simulink model "delayed_output"  (R2023b)
settings: Solver=VariableStepAuto  StartTime=0.0  StopTime=10.0  FixedStep=0.002  RelTol=1e-3
libraries: simulink x1
settings Model: Creator=franc  LastModifiedBy=franc

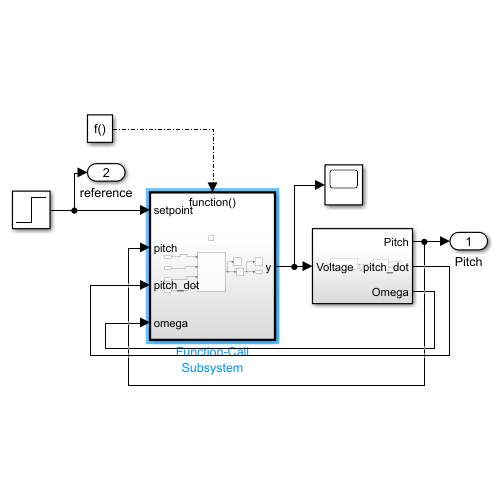
[thumbnail: Simulink's stored preview of the top-level diagram]
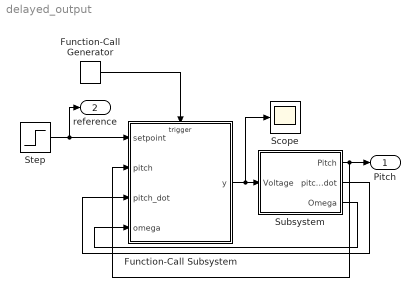
== system delayed_output ==
  Function-Call Generator : simulink/Ports & Subsystems/Function-Call Generator  sample_time=0.1  numberOfIterations=1  DisallowWideOutput=off
  Function-Call Subsystem : Subsystem  TreatAsAtomicUnit=on
  Scope : Scope
  Step : Step  SampleTime=0
  Subsystem : Subsystem
  Pitch : Outport
  reference : Outport  Port=2
  wires:
  Function-Call Generator/1 -> Function-Call Subsystem/Trigger
  Step/1 -> reference/1, Function-Call Subsystem/1(setpoint)
  Function-Call Subsystem/1(y) -> Scope/1, Subsystem/1(Voltage)
  Subsystem/2(pitch_dot) -> Function-Call Subsystem/3(pitch_dot)
  Subsystem/3(Omega) -> Function-Call Subsystem/4(omega)
  Subsystem/1(Pitch) -> Pitch/1, Function-Call Subsystem/2(pitch)

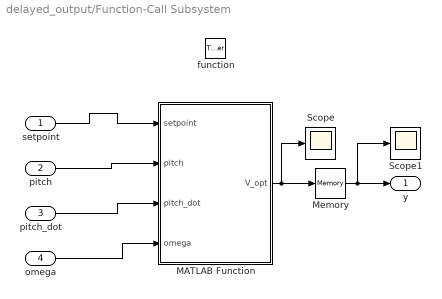
== system delayed_output/Function-Call Subsystem ==
  setpoint : Inport
  pitch : Inport  Port=2
  pitch_dot : Inport  Port=3
  omega : Inport  Port=4
  function : TriggerPort  TriggerType=function-call  VariantControl=(inherit)  SampleTimeType=periodic  SampleTime=0.1
  MATLAB Function : MATLAB Function  TreatAsAtomicUnit=on
  Memory : Memory  InheritSampleTime=on
  Scope : Scope
  Scope1 : Scope
  y : Outport
  wires:
  setpoint/1 -> MATLAB Function/1(setpoint)
  MATLAB Function/1(V_opt) -> Scope/1, Memory/1
  pitch/1 -> MATLAB Function/2(pitch)
  pitch_dot/1 -> MATLAB Function/3(pitch_dot)
  omega/1 -> MATLAB Function/4(omega)
  Memory/1 -> Scope1/1, y/1

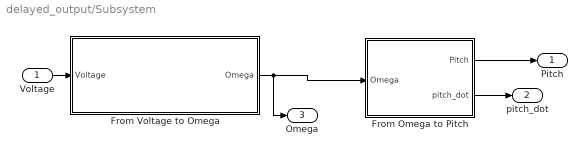
== system delayed_output/Subsystem ==
  Voltage : Inport
  From Omega to Pitch : Subsystem
  From Voltage to Omega : Subsystem
  Pitch : Outport
  pitch_dot : Outport  Port=2
  Omega : Outport  Port=3
  wires:
  From Voltage to Omega/1(Omega) -> Omega/1, From Omega to Pitch/1(Omega)
  Voltage/1 -> From Voltage to Omega/1(Voltage)
  From Omega to Pitch/1(Pitch) -> Pitch/1
  From Omega to Pitch/2(pitch_dot) -> pitch_dot/1

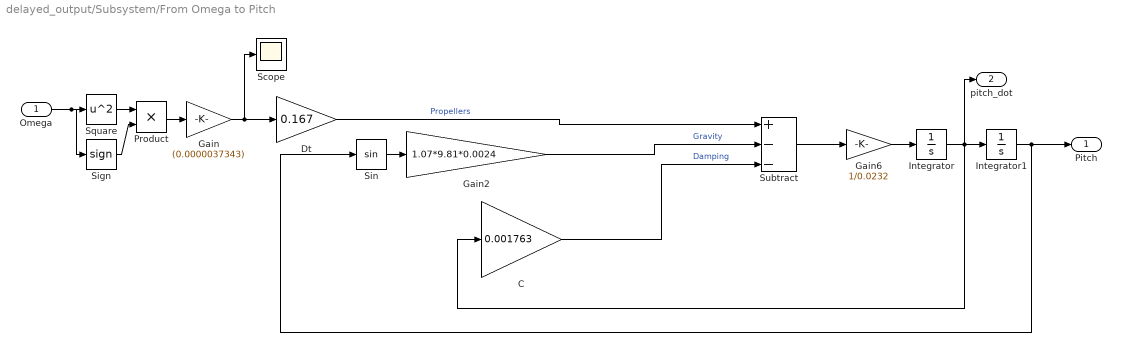
== system delayed_output/Subsystem/From Omega to Pitch ==
  Omega : Inport
  C : Gain  Gain=0.001763
  Dt : Gain  Gain=0.167
  Gain : Gain  Gain=(0.0000037343)
  Gain2 : Gain  Gain=1.07*9.81*0.0024
  Gain6 : Gain  Gain=1/0.0232
  Integrator : Integrator
  Integrator1 : Integrator
  Product : Product
  Scope : Scope
  Sign : Signum  ZeroCross=off
  Sin : Trigonometry
  Square : Math  Operator=square
  Subtract : Sum  Inputs=+--
  Pitch : Outport
  pitch_dot : Outport  Port=2
  wires:
  Integrator1/1 -> Pitch/1, Sin/1
  Sin/1 -> Gain2/1
  Subtract/1 -> Gain6/1
  Gain2/1 -> Subtract/2  "Gravity"
  C/1 -> Subtract/3  "Damping"
  Omega/1 -> Sign/1, Square/1
  Gain6/1 -> Integrator/1
  Integrator/1 -> pitch_dot/1, Integrator1/1, C/1
  Dt/1 -> Subtract/1  "Propellers"
  Product/1 -> Gain/1
  Square/1 -> Product/1
  Sign/1 -> Product/2
  Gain/1 -> Scope/1, Dt/1

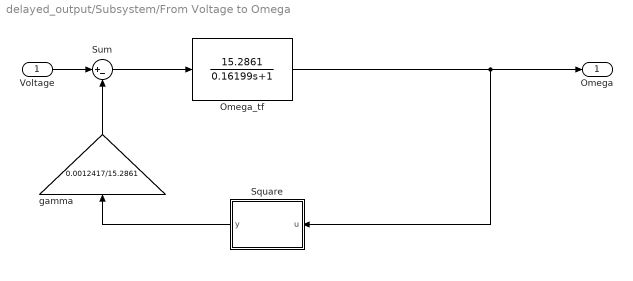
== system delayed_output/Subsystem/From Voltage to Omega ==
  Voltage : Inport
  Omega_tf : TransferFcn  Numerator=15.2861  Denominator=[0.16199 1]
  Square : MATLAB Function  TreatAsAtomicUnit=on
  Sum : Sum  Inputs=|+-
  gamma : Gain  Gain=0.0012417/15.2861
  Omega : Outport
  wires:
  Voltage/1 -> Sum/1
  gamma/1 -> Sum/2
  Square/1(y) -> gamma/1
  Omega_tf/1 -> Omega/1, Square/1(u)
  Sum/1 -> Omega_tf/1

== matlab function delayed_output/Function-Call Subsystem/MATLAB Function ==
  data: setpoint input size=1; V_opt output size=1; pitch input size=1; pitch_dot input size=1; omega input size=1
function V_opt = asyncFunction(setpoint,pitch,pitch_dot,omega)
    fun=@(V)simulate_pitch(0.1,[omega,pitch_dot,pitch],V,setpoint);
    opts=optimoptions("fmincon","Algorithm","sqp","MaxFunctionEvaluations",1e5);
    size=10;
    V_opt_full=fmincon(fun,1*ones(size,1),[eye(size);-eye(size)],[16*ones(size,1);16*ones(size,1)],[],[],[],[],[],opts);
    V_opt=V_opt_full(1); 
end

== matlab function delayed_output/Subsystem/From Voltage to Omega/Square ==
  data: u input; y output
function y = fcn(u)
y=u^2*sign(u);
